simulink subsystem "MPC6_nlpsol"  (R2022b)
settings: Solver=VariableStepAuto  StartTime=0.0  StopTime=10.0  RelTol=1e-3
undefined symbols (not defined in the file): param_MPC6, param_MPC6_init_guess, param_traj_data, param_weight_init
settings Model: Creator=emu  LastModifiedBy=emu
settings OptimizationCC: ReuseModelBlockBuffer=on

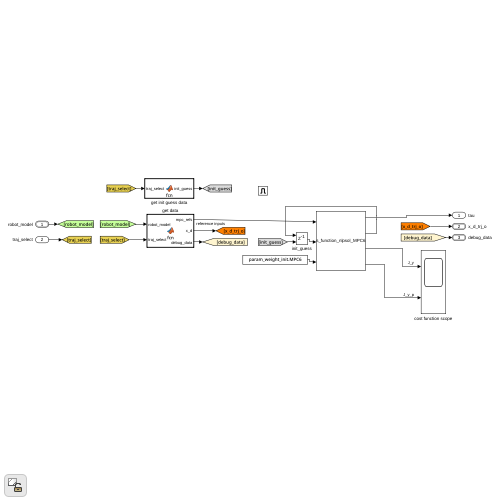
[thumbnail: Simulink's stored preview of the top-level diagram]
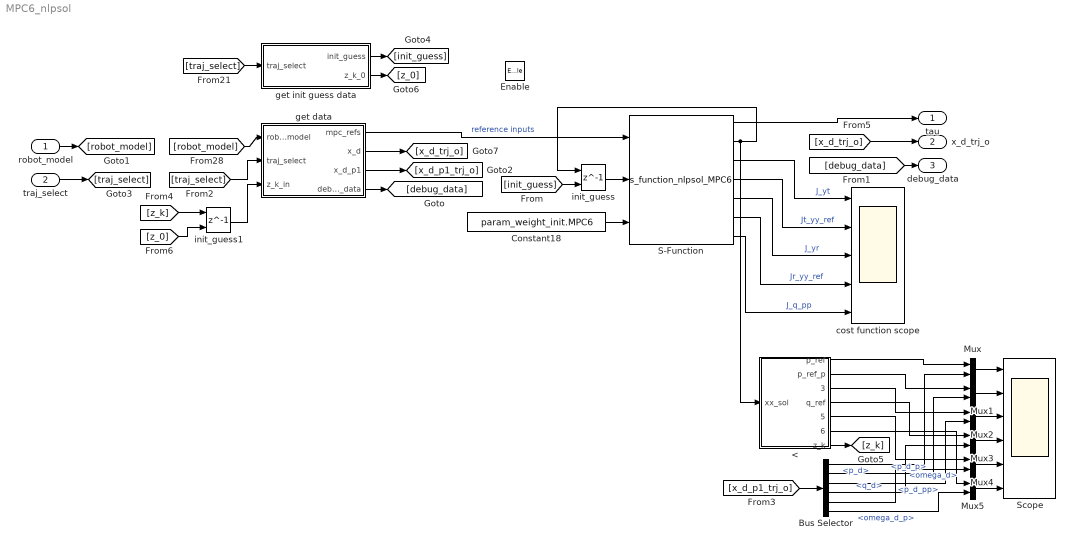
== system MPC6_nlpsol ==
  robot_model : Inport  OutDataTypeStr=Bus: robot_model
  traj_select : Inport  Port=2
  Enable : EnablePort
  < : MATLAB Function  TreatAsAtomicUnit=on
  Bus Selector : BusSelector  OutputSignals=p_d,p_d_p,p_d_pp,q_d,omega_d,omega_d_p
  Constant18 : Constant  Value=param_weight_init.MPC6  VectorParams1D=off
  Mux{,1..5} (6 alike) : Mux  Inputs=2
  S-Function : S-Function  FunctionName=s_function_nlpsol_MPC6  Parameters='s_functions/fr3_6dof/MPC6.casadi', 'MPC6'  SFunctionModules='MPC6'  SFunctionDeploymentMode=off  EnableBusSupport=off
  Scope : Scope  NumInputPorts=6
  cost function scope : Scope  NumInputPorts=5
  get data : MATLAB Function  TreatAsAtomicUnit=on
  get init guess data : MATLAB Function  TreatAsAtomicUnit=on
  init_guess : Delay  DelayLength=1  InitialConditionSource=Input port  InitialCondition=1
      settings: InputPortMap=u0,p4
  init_guess1 : Delay  DelayLength=1  InitialConditionSource=Input port  InitialCondition=1
      settings: InputPortMap=u0,p4
  tau : Outport
  x_d_trj_o : Outport  Port=2  OutDataTypeStr=Bus: x_d
  debug_data : Outport  Port=3  OutDataTypeStr=Bus: debug_data_bus
  wires:
  get init guess data/2(z_k_0) -> [z_0]
  [z_0] -> init_guess1/2
  init_guess1/1 -> get data/3(z_k_in)
  [z_k] -> init_guess1/1
  </7(z_k) -> [z_k]
  get data/3(x_d_p1) -> [x_d_p1_trj_o]
  Bus Selector/6 -> Mux5/2  "<omega_d_p>"
  </6(omega_ref_p) -> Mux5/1
  Bus Selector/5 -> Mux4/2  "<omega_d>"
  </5(omega_ref) -> Mux4/1
  Bus Selector/4 -> Mux3/2  "<q_d>"
  </4(q_ref) -> Mux3/1
  Bus Selector/3 -> Mux2/2  "<p_d_pp>"
  </3(p_ref_pp) -> Mux2/1
  Bus Selector/2 -> Mux1/2  "<p_d_p>"
  </2(p_ref_p) -> Mux1/1
  Bus Selector/1 -> Mux/2  "<p_d>"
  </1(p_ref) -> Mux/1
  Mux5/1 -> Scope/6
  Mux4/1 -> Scope/5
  Mux3/1 -> Scope/4
  Mux2/1 -> Scope/3
  Mux1/1 -> Scope/2
  Mux/1 -> Scope/1
  [x_d_p1_trj_o] -> Bus Selector/1
  S-Function/7 -> cost function scope/5  "J_q_pp"
  S-Function/6 -> cost function scope/4  "Jr_yy_ref"
  S-Function/4 -> cost function scope/2  "Jt_yy_ref"
  S-Function/5 -> cost function scope/3  "J_yr"
  Constant18/1 -> S-Function/3
  S-Function/3 -> cost function scope/1  "J_yt"
  [x_d_trj_o] -> x_d_trj_o/1
  robot_model/1 -> [robot_model]
  get data/4(debug_data) -> [debug_data]
  get data/2(x_d) -> [x_d_trj_o]
  S-Function/1 -> tau/1
  traj_select/1 -> [traj_select]
  [traj_select] -> get init guess data/1(traj_select)
  get data/1(mpc_refs) -> S-Function/1  "reference inputs"
  init_guess/1 -> S-Function/2
  [debug_data] -> debug_data/1
  S-Function/2 -> init_guess/1, </1(xx_sol)
  [robot_model] -> get data/1(robot_model)
  [traj_select] -> get data/2(traj_select)
  get init guess data/1(init_guess) -> [init_guess]
  [init_guess] -> init_guess/2

== matlab function MPC6_nlpsol/get data ==
  settings: updateMethod=DISCRETE  sampleTime=param_global.Ta
  data: mpc_refs output; robot_model input Bus: robot_model; param_MPC6 parameter; x_d output Bus: x_d; x_d_p1 output Bus: x_d; debug_data output Bus: debug_data_bus; param_traj_data parameter; traj_select input; z_k_in input
function [mpc_refs, x_d, x_d_p1, debug_data] = fcn(robot_model, param_MPC6, param_traj_data, traj_select, z_k_in)
persistent cnt;

if(isempty(cnt))
    cnt = 1;
end

param_MPC = param_MPC6;
N         = param_MPC.N;
N_step    = param_MPC.N_step;

% Parameters
q    = robot_model.q;      % generalized coordinates
q_p  = robot_model.q_p;  % time derivative of generalized coordinates
q_pp = robot_model.q_pp;
H    = robot_model.H;
J    = robot_model.J;
J_p  = robot_model.J_p;

R = H(1:3,1:3);% desired Orientation as rotational matrix
R_d = param_traj_data.R_d(:,:, cnt, traj_select);
q_d = param_traj_data.q_d(:, cnt, traj_select);

%y_q_err = quat_mult(y_q_e, quat_inv(param_traj_data.q_d(1:4, cnt, traj_select)));
q_err = rotation2quaternion(R*R_d');
%y_q_e = rotation2quaternion(R);
q_e = quat_mult(q_d, q_err);

% Current Pose of Endeffector
y = [H(1:3,4); q_e];
y_p = J*q_p;
y_pp = J*q_pp + J_p*q_p;



x_k = [q;q_p];

% Assemble vector of recieved output measurements
p_d    = param_traj_data.p_d(   1:3, cnt : N_step : cnt + (N)*N_step, traj_select);
p_d_p  = param_traj_data.p_d_p( 1:3, cnt : N_step : cnt + (N)*N_step, traj_select);
p_d_pp = param_traj_data.p_d_pp(1:3, cnt : N_step : cnt + (N)*N_step, traj_select);

% RPY XYZ angles
Phi_d = param_traj_data.Phi_d(      1:3, cnt : N_step : cnt + (N) * N_step, traj_select ); % (Phi_0 ... Phi_N)
Phi_d_p = param_traj_data.Phi_d_p(  1:3, cnt : N_step : cnt + (N) * N_step, traj_select ); % (Phi_p_0 ... Phi_p_N)
Phi_d_pp = param_traj_data.Phi_d_pp(1:3, cnt : N_step : cnt + (N) * N_step, traj_select ); % (Phi_pp_0 ... Phi_pp_N)

q_d    = param_traj_data.q_d(      1:4, cnt : N_step : cnt + (N)*N_step, traj_select);
q_d_p  = param_traj_data.q_d_p(    1:4, cnt : N_step : cnt + (N)*N_step, traj_select);
q_d_pp = param_traj_data.q_d_pp(   1:4, cnt : N_step : cnt + (N)*N_step, traj_select);

omega_d   = param_traj_data.omega_d(  1:3, cnt : N_step : cnt + (N)*N_step, traj_select);
omega_d_p = param_traj_data.omega_d_p(1:3, cnt : N_step : cnt + (N)*N_step, traj_select);

alpha_d    = param_traj_data.alpha_d(           :, cnt : N_step : cnt + (N)*N_step, traj_select);
alpha_d_p  = param_traj_data.alpha_d_p(         :, cnt : N_step : cnt + (N)*N_step, traj_select);
alpha_d_pp = param_traj_data.alpha_d_pp(        :, cnt : N_step : cnt + (N)*N_step, traj_select);
rot_ax_d   = param_traj_data.rot_ax_d(          :, cnt : N_step : cnt + (N)*N_step, traj_select);
alpha_d_offset = param_traj_data.alpha_d_offset(:, cnt : N_step : cnt + (N)*N_step, traj_select);
q_d_rel = param_traj_data.q_d_rel(              :, cnt : N_step : cnt + (N)*N_step, traj_select);


alpha_var = 4;
if(alpha_var == 1) % only alpha ref with fixed rot ax
    y_d = [p_d; alpha_d; rot_ax_d; alpha_d_offset; q_d_rel];
    y_d_p = [p_d_p; alpha_d_p];
    y_d_pp = [p_d_pp; alpha_d_pp];
    z_k = [y_d(1:3,1); y_d_p(1:3,1); y_d(4,1); y_d_p(4,1)]; % [p_d_0; p_d_p_0; alpha_d_0; alpha_d_p_0]
elseif(alpha_var == 2) % full quat_ref, quat_p_ref, quat_pp_ref integration
    y_d = [p_d; q_d];
    y_d_p = [p_d_p; q_d_p];
    y_d_pp = [p_d_pp; q_d_pp];
    z_k = [y_d(1:3,1); y_d_p(1:3,1); y_d(4:7,1); y_d_p(4:7,1);]; % p_d_0, q_d_0, p_d_p_0, q_d_p_0
elseif(alpha_var == 3) %alpha == 3: euler angles ref
    y_d = [p_d; Phi_d];
    y_d_p = [p_d_p; Phi_d_p];
    y_d_pp = [p_d_pp; Phi_d_pp];
    z_k = [y_d(1:3,1); y_d_p(1:3,1); y_d(4:6,1); y_d_p(4:6,1);]; % p_d_0, q_d_0, p_d_p_0, q_d_p_0
else  %alpha == 4: quat omega ref
    y_d = [p_d; q_d];
    y_d_p = [p_d_p; omega_d];
    y_d_pp = [p_d_pp; omega_d_p];
    z_k = [y_d(1:3,1); y_d_p(1:3,1); y_d(4:7,1); y_d_p(4:6,1);]; % p_d_0, q_d_0, p_d_p_0, q_d_p_0
    %z_k = [y(1:3); y_p(1:3); rotation2quaternion(R); y_p(4:6);];
    %z_k = z_k_in;
end



%% Reference out
% z_0_0 = [p_d_0(:,1); q_d_0(:,1); p_d_p_0(:,1); omega_d_0(:,1)]
% z_d_init_guess_0 = [p_d_0; q_d_0; p_p_d_0; omega_d_0];
% mpc_init_reference_values = [x_0_0(:); z_0_0(:); z_d_init_guess_0(:)];

mpc_refs = [x_k(:); z_k(:); y_d(:); y_d_p(:); y_d_pp(:)];
%mpc_refs = [x_k(:); y_d(:); y_d_p(:); y_d_pp(:)];

%mpc_refs = [x_k(:); y_d(:)];
%mpc_refs = [x_k(:); Phi_d_traj(:)];

%% TRAJECTORY OUT
x_d.p_d       = param_traj_data.p_d(1:3, cnt , traj_select);    %y0
x_d.p_d_p     = param_traj_data.p_d_p(1:3, cnt , traj_select);  %y0p
x_d.p_d_pp    = param_traj_data.p_d_pp(1:3, cnt , traj_select); %y0pp
x_d.Phi_d     = param_traj_data.Phi_d(:, cnt , traj_select);
x_d.Phi_d_p   = param_traj_data.Phi_d_p(:, cnt, traj_select);
x_d.Phi_d_pp  = param_traj_data.Phi_d_pp(:,cnt, traj_select);
x_d.R_d       = R_d;
x_d.q_d       = q_d(1:4, 1);
x_d.q_d_p     = param_traj_data.q_d_p(1:4, cnt, traj_select);
x_d.q_d_pp    = param_traj_data.q_d_pp(1:4, cnt, traj_select);
x_d.omega_d   = omega_d(1:3, 1);
x_d.omega_d_p = omega_d_p(1:3, 1);
x_d.alpha_d    = alpha_d(:, 1);
x_d.alpha_d_p  = alpha_d_p(:, 1);
x_d.alpha_d_pp = alpha_d_pp(:, 1);
x_d.rot_ax_d   = rot_ax_d(:, 1);
x_d.alpha_d_offset = alpha_d_offset(:, 1);
x_d.q_d_rel = q_d_rel(:, 1);

%% TRAJECTORYp1 OUT
x_d_p1.p_d       = param_traj_data.p_d(1:3, cnt+1 , traj_select);    %y0
x_d_p1.p_d_p     = param_traj_data.p_d_p(1:3, cnt+1 , traj_select);  %y0p
x_d_p1.p_d_pp    = param_traj_data.p_d_pp(1:3, cnt+1 , traj_select); %y0pp
x_d_p1.Phi_d     = param_traj_data.Phi_d(:, cnt+1 , traj_select);
x_d_p1.Phi_d_p   = param_traj_data.Phi_d_p(:, cnt+1, traj_select);
x_d_p1.Phi_d_pp  = param_traj_data.Phi_d_pp(:,cnt+1, traj_select);
x_d_p1.R_d       = R_d;
x_d_p1.q_d       = q_d(1:4, 2);
x_d_p1.q_d_p     = param_traj_data.q_d_p(1:4, cnt+1, traj_select);
x_d_p1.q_d_pp    = param_traj_data.q_d_pp(1:4, cnt+1, traj_select);
x_d_p1.omega_d   = omega_d(1:3, 2);
x_d_p1.omega_d_p = omega_d_p(1:3, 2);
x_d_p1.alpha_d    = alpha_d(:, 2);
x_d_p1.alpha_d_p  = alpha_d_p(:, 2);
x_d_p1.alpha_d_pp = alpha_d_pp(:, 2);
x_d_p1.rot_ax_d   = rot_ax_d(:, 2);
x_d_p1.alpha_d_offset = alpha_d_offset(:, 2);
x_d_p1.q_d_rel = q_d_rel(:, 2);

%% DEBUG
debug_data.p           = y(1:3);
debug_data.p_p         = y_p(1:3);
debug_data.p_pp        = y_pp(1:3);
debug_data.Phi     = rotm2eul_v2(R);
debug_data.Phi_p   = [0; 0; 0]; % ??????
debug_data.Phi_pp  = [0; 0; 0]; % ??????
debug_data.q           = y(4:7);
debug_data.omega       = y_p(4:6);
debug_data.omega_p     = y_pp(4:6);
debug_data.p_err       = y(1:3) - param_traj_data.p_d(:, cnt, traj_select);
debug_data.p_p_err     = y_p(1:3) - param_traj_data.p_d_p(:, cnt, traj_select);
debug_data.p_pp_err    = y_pp(1:3) - param_traj_data.p_d_pp(:, cnt, traj_select);
debug_data.q_err       = q_err;
debug_data.omega_err   = y_p(4:6)  - omega_d(1:3, 1);
debug_data.omega_p_err = y_pp(4:6) - omega_d_p(1:3, 1);

cnt = cnt+1;

== matlab function MPC6_nlpsol/get init guess data ==
  data: traj_select input; param_MPC6_init_guess parameter; init_guess output; param_traj_data parameter; z_k_0 output
function [init_guess, z_k_0]  = fcn(traj_select, param_MPC6_init_guess, param_traj_data)

%init_guess = param_MPC6_init_guess.init_guess(1,:);
init_guess = param_MPC6_init_guess.init_guess(traj_select,:);

p_d    = param_traj_data.p_d(   1:3, 1, traj_select);
p_d_p  = param_traj_data.p_d_p( 1:3, 1, traj_select);

q_d    = param_traj_data.q_d(      1:4, 1, traj_select);
omega_d   = param_traj_data.omega_d(  1:3, 1, traj_select);
z_k_0 = [p_d; p_d_p; q_d; omega_d];

== matlab function MPC6_nlpsol/< ==
  data: xx_sol input; p_ref output; param_MPC6 parameter; p_ref_p output; p_ref_pp output; q_ref output; omega_ref output; omega_ref_p output; z_k output
function [p_ref, p_ref_p, p_ref_pp, q_ref, omega_ref, omega_ref_p, z_k] = fcn(xx_sol, param_MPC6)

param_MPC = param_MPC6;

pp_indices = param_MPC.pp;
pp_dim = param_MPC.pp_dim;

rr_indices = param_MPC.rr;
rr_dim = param_MPC.rr_dim;

pp = reshape(xx_sol(pp_indices), pp_dim);
rr = reshape(xx_sol(rr_indices), rr_dim);

p_ref = pp(1:3, 1 + (1));
p_ref_p = pp(4:6, 1 + (1));
p_ref_pp = pp(7:9, 1 + (1));

q_ref = rr(1:4, 1 + (1));
omega_ref = rr(5:7, 1 + (1));
omega_ref_p = rr(8:10, 1 + (1));

z_k = [p_ref; p_ref_p; q_ref; omega_ref];
